simulink model "R2_double"  (R2014b)
settings: Solver=ode3  SolverMode=SingleTasking  StartTime=0.0  StopTime=Tsim  FixedStep=Ts  RelTol=1e-3
InitFcn:
  | configDoubleIntegrator
libraries: simulink x1
settings Model: CovMetricSettings=dwe  CovHtmlReporting=off  covSaveCumulativeToWorkspaceVar=off  CovSaveSingleToWorkspaceVar=off  CovExternalEMLEnable=on  CovSFcnEnable=on  Creator=mnade  LastModifiedBy=nina
settings DataIOCC: LimitDataPoints=off  SaveFormat=StructureWithTime
settings DebuggingCC: SolverPrmCheckMsg=none  FrameProcessingCompatibilityMsg=error  SFUnexpectedBacktrackingDiag=error  SFNoUnconditionalDefaultTransitionDiag=error
settings HardwareCC: ProdBitPerPointer=64  ProdLargestAtomicFloat=Float  ProdIntDivRoundTo=Zero  ProdEndianess=LittleEndian  ProdHWDeviceType=Specified
settings ModelReferenceCC: PropagateSignalLabelsOutOfModel=on
settings GRTTargetCC: TargetLangStandard=C99 (ISO)  GeneratePreprocessorConditionals=Use local settings

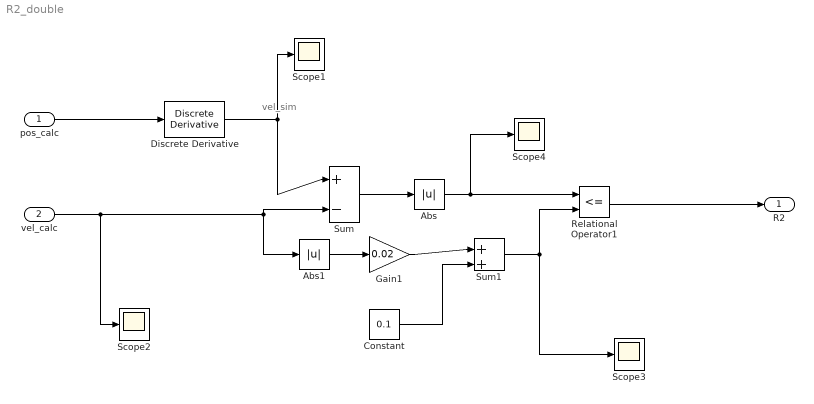
== system R2_double ==
  note: vel_sim
  pos_calc : Inport
  vel_calc : Inport  Port=2
  Abs : Abs
  Abs1 : Abs
  Constant : Constant  Value=0.1
  Discrete Derivative : simulink/Discrete/Discrete Derivative  gainval=1.0  ICPrevScaledInput=0.0  InputProcessing=Inherited  OutMin=[]  OutMax=[]  OutDataType=fixdt(1, 16)  OutScaling=2^-10  DoSatur=off
  Gain1 : Gain  Gain=0.02
  Relational Operator1 : RelationalOperator  Operator=<=  OutDataTypeStr=boolean
  Scope{1..4} (4 alike) : Scope
      Scope3 settings: SaveName=ScopeData2
      Scope4 settings: SaveName=ScopeData3
  Sum : Sum  Inputs=|+-
  Sum1 : Sum  Inputs=|++
  R2 : Outport
  wires:
  pos_calc/1 -> Discrete Derivative/1
  Relational Operator1/1 -> R2/1
  Discrete Derivative/1 -> Sum/1, Scope1/1
  vel_calc/1 -> Scope2/1, Abs1/1, Sum/2
  Sum/1 -> Abs/1
  Abs/1 -> Scope4/1, Relational Operator1/1
  Abs1/1 -> Gain1/1
  Sum1/1 -> Scope3/1, Relational Operator1/2
  Gain1/1 -> Sum1/1
  Constant/1 -> Sum1/2
